simulink model "Lab6"  (R2018a)
settings: Solver=VariableStepAuto  StartTime=0.0  StopTime=10.0  RelTol=1e-3
settings Model: Creator=Salman Prottoy  LastModifiedBy=Salman Prottoy

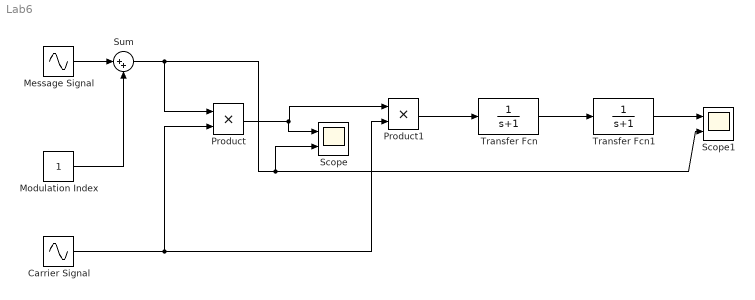
== system Lab6 ==
  "Carrier Signal " : Sin  Frequency=2*pi*25  SampleTime=1/5000
  "Message Signal " : Sin  Frequency=2*pi  SampleTime=1/5000
  "Modulation Index " : Constant
  "Product " : Product
  "Product1 " : Product
  "Scope " : Scope  NumInputPorts=2
  "Scope1 " : Scope  NumInputPorts=2
  Sum : Sum  Inputs=|++
  "Transfer Fcn " : TransferFcn  Denominator=[1 1]
  "Transfer Fcn1 " : TransferFcn  Denominator=[1 1]
  wires:
  "Message Signal "/1 -> Sum/1
  "Modulation Index "/1 -> Sum/2
  "Carrier Signal "/1 -> "Product "/2, "Product1 "/2
  Sum/1 -> "Scope1 "/2, "Scope "/2, "Product "/1
  "Product "/1 -> "Product1 "/1, "Scope "/1
  "Product1 "/1 -> "Transfer Fcn "/1
  "Transfer Fcn "/1 -> "Transfer Fcn1 "/1
  "Transfer Fcn1 "/1 -> "Scope1 "/1
